simulink model "VM_22042020"  (R2019b)
settings: Solver=VariableStepAuto  StartTime=0.0  StopTime=120  RelTol=1e-3
libraries: aerolibconvert2 x3, simulink x2
settings Model: Creator=diego  LastModifiedBy=diego
settings DataIOCC: OutputOption=SpecifiedOutputTimes  OutputTimes=[0:0.0001:120]

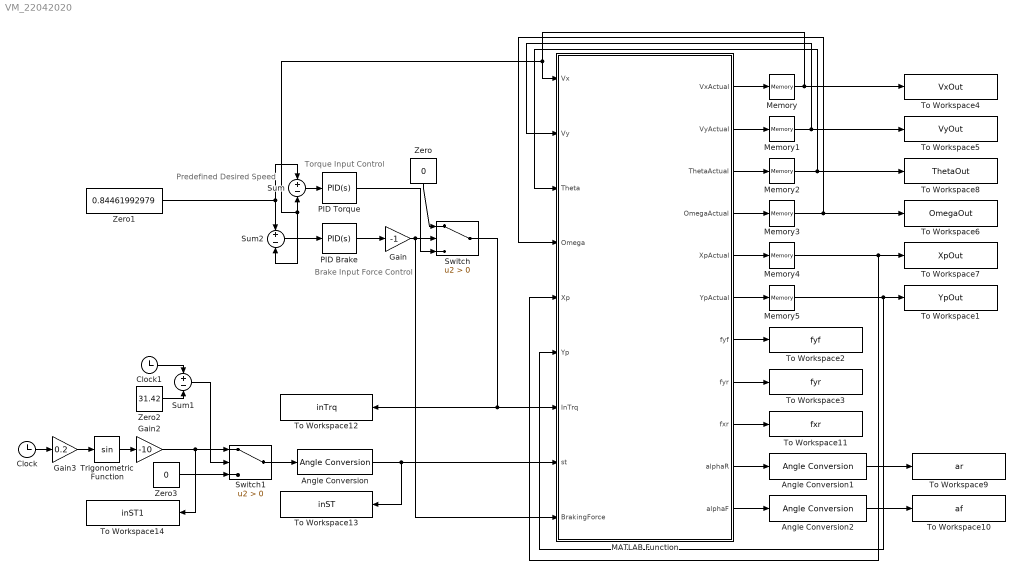
== system VM_22042020 ==
  note: Brake Input Force Control
  note: Torque Input Control
  note: Predefined Desired Speed
  Angle Conversion : aerolibconvert2/Angle Conversion  IU=deg  OU=rad
  Angle Conversion1 : aerolibconvert2/Angle Conversion  IU=rad  OU=deg
  Angle Conversion2 : aerolibconvert2/Angle Conversion  IU=rad  OU=deg
  Clock : Clock
  Clock1 : Clock
  Gain : Gain  Gain=-1
  Gain2 : Gain  Gain=-10
  Gain3 : Gain  Gain=0.2
  MATLAB Function : MATLAB Function  TreatAsAtomicUnit=on
  Memory{,1..5} (6 alike) : Memory
  PID Brake : simulink/Continuous/PID Controller  Controller=PID  Form=Parallel  TimeDomain=Continuous-time  SampleTime=-1  IntegratorMethod=Forward Euler  FilterMethod=Forward Euler  ControllerParametersSource=internal  P=7  I=0.28  D=0.5  UseFilter=on  N=100  TunerSelectOption=Transfer Function Based (PID Tuner App)  InitialConditionSource=internal  InitialConditionForIntegrator=0  InitialConditionForFilter=0  DifferentiatorICPrevScaledInput=0  ExternalReset=none  TrackingMode=off  Kt=1  LimitOutput=on  UpperSaturationLimit=0  LowerSaturationLimit=-10000  LinearizeAsGain=on  AntiWindupMode=none  Kb=1  POutMin=[]  POutMax=[]  IOutMin=[]  IOutMax=[]  DOutMin=[]  DOutMax=[]  NOutMin=[]  NOutMax=[]  SumOutMin=[]  SumOutMax=[]  SaturationOutMin=[]  SaturationOutMax=[]  PParamMin=[]  PParamMax=[]  IParamMin=[]  IParamMax=[]  DParamMin=[]  DParamMax=[]  NParamMin=[]  NParamMax=[]  KbParamMin=[]  KbParamMax=[]  KtParamMin=[]  KtParamMax=[]  KbOutMin=[]  KbOutMax=[]  KtOutMin=[]  KtOutMax=[]  IntegratorOutMin=[]  IntegratorOutMax=[]  FilterOutMin=[]  FilterOutMax=[]  SumI1OutMin=[]  SumI1OutMax=[]  SumI2OutMin=[]  SumI2OutMax=[]  SumI3OutMin=[]  SumI3OutMax=[]  SumI4OutMin=[]  SumI4OutMax=[]  SumDOutMin=[]  SumDOutMax=[]  DifferentiatorOutMin=[]  DifferentiatorOutMax=[]  FilterDiffOutCoefMin=[]  FilterDiffOutCoefMax=[]  ReciprocalOutMin=[]  ReciprocalOutMax=[]  SumDenOutMin=[]  SumDenOutMax=[]  SumNumOutMin=[]  SumNumOutMax=[]  DivideOutMin=[]  DivideOutMax=[]  IntegratorContinuousStateAttributes=''  IntegratorStateMustResolveToSignalObject=off  IntegratorRTWStateStorageClass=Auto  FilterContinuousStateAttributes=''  FilterStateMustResolveToSignalObject=off  FilterRTWStateStorageClass=Auto  ParallelPVariant=InternalParameters  IdealPVariant=Disabled  IVariant=InternalParameters  DVariant=InternalParameters  IntegratorVariant=Continuous  SatVariant=Enabled  AWVariant=Passthrough  PCopyVariant=Disabled  TRVariant=Disabled  FdbkBlocksVariant=Forward  IdealPFdbkVariant=Disabled  SatFdbkVariant=Disabled  DerivativeFilterVariant=ContFilter  NVariant=InternalParameters  NCopyVariant=Disabled  FilterICVariant=InternalICsFilter  IntegratorICVariant=InternalICs  ExternalResetVariant=Disabled  TRSumVariant=Passthrough  SumFdbkVariant=Disabled  SumVariant=Sum_PID
  PID Torque : simulink/Continuous/PID Controller  Controller=PID  Form=Parallel  TimeDomain=Continuous-time  SampleTime=-1  IntegratorMethod=Forward Euler  FilterMethod=Forward Euler  ControllerParametersSource=internal  P=12  I=0.5  D=0.5  UseFilter=on  N=100  TunerSelectOption=Transfer Function Based (PID Tuner App)  InitialConditionSource=internal  InitialConditionForIntegrator=0  InitialConditionForFilter=0  DifferentiatorICPrevScaledInput=0  ExternalReset=none  TrackingMode=off  Kt=1  LimitOutput=on  UpperSaturationLimit=120  LowerSaturationLimit=0  LinearizeAsGain=on  AntiWindupMode=none  Kb=1  POutMin=[]  POutMax=[]  IOutMin=[]  IOutMax=[]  DOutMin=[]  DOutMax=[]  NOutMin=[]  NOutMax=[]  SumOutMin=[]  SumOutMax=[]  SaturationOutMin=[]  SaturationOutMax=[]  PParamMin=[]  PParamMax=[]  IParamMin=[]  IParamMax=[]  DParamMin=[]  DParamMax=[]  NParamMin=[]  NParamMax=[]  KbParamMin=[]  KbParamMax=[]  KtParamMin=[]  KtParamMax=[]  KbOutMin=[]  KbOutMax=[]  KtOutMin=[]  KtOutMax=[]  IntegratorOutMin=[]  IntegratorOutMax=[]  FilterOutMin=[]  FilterOutMax=[]  SumI1OutMin=[]  SumI1OutMax=[]  SumI2OutMin=[]  SumI2OutMax=[]  SumI3OutMin=[]  SumI3OutMax=[]  SumI4OutMin=[]  SumI4OutMax=[]  SumDOutMin=[]  SumDOutMax=[]  DifferentiatorOutMin=[]  DifferentiatorOutMax=[]  FilterDiffOutCoefMin=[]  FilterDiffOutCoefMax=[]  ReciprocalOutMin=[]  ReciprocalOutMax=[]  SumDenOutMin=[]  SumDenOutMax=[]  SumNumOutMin=[]  SumNumOutMax=[]  DivideOutMin=[]  DivideOutMax=[]  IntegratorContinuousStateAttributes=''  IntegratorStateMustResolveToSignalObject=off  IntegratorRTWStateStorageClass=Auto  FilterContinuousStateAttributes=''  FilterStateMustResolveToSignalObject=off  FilterRTWStateStorageClass=Auto  ParallelPVariant=InternalParameters  IdealPVariant=Disabled  IVariant=InternalParameters  DVariant=InternalParameters  IntegratorVariant=Continuous  SatVariant=Enabled  AWVariant=Passthrough  PCopyVariant=Disabled  TRVariant=Disabled  FdbkBlocksVariant=Forward  IdealPFdbkVariant=Disabled  SatFdbkVariant=Disabled  DerivativeFilterVariant=ContFilter  NVariant=InternalParameters  NCopyVariant=Disabled  FilterICVariant=InternalICsFilter  IntegratorICVariant=InternalICs  ExternalResetVariant=Disabled  TRSumVariant=Passthrough  SumFdbkVariant=Disabled  SumVariant=Sum_PID
  Sum : Sum  Inputs=+-
  Sum1 : Sum  Inputs=+-
  Sum2 : Sum  Inputs=+-
  Switch : Switch  Criteria=u2 > Threshold
  Switch1 : Switch  Criteria=u2 > Threshold
  To Workspace1 : ToWorkspace  VariableName=YpOut  SaveFormat=Timeseries  SampleTime=-1
  To Workspace10 : ToWorkspace  VariableName=af  SaveFormat=Timeseries  SampleTime=-1
  To Workspace11 : ToWorkspace  VariableName=fxr  SaveFormat=Timeseries  SampleTime=-1
  To Workspace12 : ToWorkspace  VariableName=inTrq  SaveFormat=Timeseries  SampleTime=-1
  To Workspace13 : ToWorkspace  VariableName=inST  SaveFormat=Timeseries  SampleTime=-1
  To Workspace14 : ToWorkspace  VariableName=inST1  SaveFormat=Timeseries  SampleTime=-1
  To Workspace2 : ToWorkspace  VariableName=fyf  SaveFormat=Timeseries  SampleTime=-1
  To Workspace3 : ToWorkspace  VariableName=fyr  SaveFormat=Timeseries  SampleTime=-1
  To Workspace4 : ToWorkspace  VariableName=VxOut  SaveFormat=Timeseries  SampleTime=-1
  To Workspace5 : ToWorkspace  VariableName=VyOut  SaveFormat=Timeseries  SampleTime=-1
  To Workspace6 : ToWorkspace  VariableName=OmegaOut  SaveFormat=Timeseries  SampleTime=-1
  To Workspace7 : ToWorkspace  VariableName=XpOut  SaveFormat=Timeseries  SampleTime=-1
  To Workspace8 : ToWorkspace  VariableName=ThetaOut  SaveFormat=Timeseries  SampleTime=-1
  To Workspace9 : ToWorkspace  VariableName=ar  SaveFormat=Timeseries  SampleTime=-1
  Trigonometric Function : Trigonometry
  Zero : Constant  Value=0  OutDataTypeStr=Inherit: Inherit via back propagation
  Zero1 : Constant  Value=0.84461992979  OutDataTypeStr=Inherit: Inherit via back propagation
  Zero2 : Constant  Value=31.42  OutDataTypeStr=Inherit: Inherit via back propagation
  Zero3 : Constant  Value=0  OutDataTypeStr=Inherit: Inherit via back propagation
  wires:
  MATLAB Function/1(VxActual) -> Memory/1
  MATLAB Function/2(VyActual) -> Memory1/1
  MATLAB Function/3(ThetaActual) -> Memory2/1
  MATLAB Function/4(OmegaActual) -> Memory3/1
  MATLAB Function/5(XpActual) -> Memory4/1
  MATLAB Function/6(YpActual) -> Memory5/1
  Memory/1 -> To Workspace4/1, Sum2/2, Sum/2, MATLAB Function/1(Vx)
  Memory1/1 -> To Workspace5/1, MATLAB Function/2(Vy)
  Memory2/1 -> To Workspace8/1, MATLAB Function/3(Theta)
  Memory3/1 -> To Workspace6/1, MATLAB Function/4(Omega)
  Memory4/1 -> MATLAB Function/5(Xp), To Workspace7/1
  Memory5/1 -> MATLAB Function/6(Yp), To Workspace1/1
  Sum/1 -> PID Torque/1
  PID Brake/1 -> Gain/1
  Gain/1 -> MATLAB Function/9(BrakingForce), Switch/2
  Zero1/1 -> Sum/1, Sum2/1
  PID Torque/1 -> Switch/3
  Sum2/1 -> PID Brake/1
  Zero/1 -> Switch/1
  Switch/1 -> To Workspace12/1, MATLAB Function/7(InTrq)
  MATLAB Function/7(fyf) -> To Workspace2/1
  MATLAB Function/8(fyr) -> To Workspace3/1
  MATLAB Function/9(fxr) -> To Workspace11/1
  Angle Conversion/1 -> MATLAB Function/8(st), To Workspace13/1
  MATLAB Function/10(alphaR) -> Angle Conversion1/1
  Angle Conversion1/1 -> To Workspace9/1
  MATLAB Function/11(alphaF) -> Angle Conversion2/1
  Angle Conversion2/1 -> To Workspace10/1
  Switch1/1 -> Angle Conversion/1
  Trigonometric Function/1 -> Gain2/1
  Clock/1 -> Gain3/1
  Zero3/1 -> Switch1/3
  Gain2/1 -> To Workspace14/1, Switch1/1
  Clock1/1 -> Sum1/1
  Zero2/1 -> Sum1/2
  Sum1/1 -> Switch1/2
  Gain3/1 -> Trigonometric Function/1

== matlab function VM_22042020/MATLAB Function ==
  data: Vx input; VxActual output; Vy input; Theta input; Omega input; Xp input; Yp input; InTrq input; st input; BrakingForce input; VyActual output; ThetaActual output; OmegaActual output; XpActual output; YpActual output; fyf output; fyr output; fxr output; alphaR output; alphaF output
function [VxActual,VyActual,ThetaActual,OmegaActual,XpActual,YpActual,fyf,fyr,fxr,alphaR,alphaF] = VehicleModel(Vx,Vy,Theta,Omega,Xp,Yp,InTrq,st,BrakingForce)
%Center of gravity location from vehicle rear axle
Lf =0.669670;
%Rear axle to center of gravity distance
Lr = 0.669670;
%Total lenght
L =Lf + Lr;
%Vehicle mas 
m = 400;
%Gravity
g = 9.81;
%weight
W = g*m;
%Friction Coef.
miu = 0.9;
%height of the center of gravity
hgc = 0.38;
%Wheel r
rad = 0.2876;
%height
height = 0.4052;
%width 
w = 1.1600;
%Vehicle yaw inertia
I = 1/12 *m*(w^2+height^2);


%Force values
fxr = InTrq/rad + BrakingForce;
fxf = 0;

%The vertical force acting on a tire
fzr = (m*g*Lf)/L + (fxr*hgc)/(L);
fzf = (m*g*Lr)/L - (fxr*hgc)/(L);

%Validating initial conditions
if(Vx ==0)
    alphaR = 0;
    alphaF = 0;
else
    alphaR = (Lr*Omega-Vy)/Vx;
    alphaF = st-(Lf*Omega+Vy)/Vx;
end

if(isnan(alphaR))
    alphaR = 0;
end

if(isnan(alphaF))
    alphaF = 0;
end

C = 1.49;
B = 0.244;
E = 0;

sh =0;
sv =0;
xf = alphaF + sh;
xr = alphaR + sh;

fyf = fzf*sin( C*atan(B*xf - E*(B*xf - atan(B*xf))) ) + sv;
fyr = fzr*sin( C*atan(B*xr - E*(B*xr - atan(B*xr))) ) + sv;

%VehicleModel
VxActual = (fxf * cos(st) + fxr - fyf*sin(st))/m + Vy*Omega;
VyActual = (fyr + fyf*cos(st)+fxf*sin(st))/m - Vx*Omega;
OmegaActual = (Lf*fyf*cos(st)-Lr*fyr+Lf*fxf*sin(st))/I;
ThetaActual = Omega;
XpActual = Vx*cos(2*pi-Theta)+Vy*cos(3/4*pi-Theta);
YpActual = Vx*sin(2*pi-Theta)+Vy*sin(3/4*pi-Theta);

%Runge Kutta Fourth Order
%x0 - Theta (Yaw Angle)
%x1 - Omega (Yaw Rate)
%x2 - Lateral Velocity Vy
%x3 - Longitudinal Velocity Vx
%x4 - Global X position
%x5 - Global Y position

%Time Step
h = 0.0001;

x0 = Theta;
x1 = Omega;
x2 = Vy;
x3 = Vx;
x4 = Xp;
x5 = Yp;

k00 = h*x0dot(x1);
k10 = h*x1dot(Lf,fxf,st,Lr,fyf,fyr,I);
k20 = h*x2dot(fxf,st,fyf,fyr,x3,x1,m);
k30 = h*x3dot(fxf,fxr,fyf,st,x2,x1,m);
k40 = h*x4dot(x2,x0,x3);
k50 = h*x5dot(x2,x0,x3);

k01 = h*x0dot(x1+0.5*k10);
k11 = h*x1dot(Lf,fxf,st,Lr,fyf,fyr,I);
k21 = h*x2dot(fxf,st,fyf,fyr,x3+0.5*k30, x1+0.5*k10,m);
k31 = h*x3dot(fxf,fxr,fyf,st,x2+0.5*k20, x1+0.5*k10,m);
k41 = h*x4dot(x2+0.5*k20,x0+0.5*k00,x3+0.5*k30);
k51 = h*x5dot(x2+0.5*k20,x0+0.5*k00,x3+0.5*k30);

k02 = h*x0dot(x1+0.5*k11);
k12 = h*x1dot(Lf,fxf,st,Lr,fyf,fyr,I);
k22 = h*x2dot(fxf,st,fyf,fyr,x3+0.5*k31, x1+0.5*k11,m);
k32 = h*x3dot(fxf,fxr,fyf,st,x2+0.5*k21, x1+0.5*k11,m);
k42 = h*x4dot(x2+0.5*k21,x0+0.5*k01,x3+0.5*k31);
k52 = h*x5dot(x2+0.5*k21,x0+0.5*k01,x3+0.5*k31);

k03 = h*x0dot(x1+k12);
k13 = h*x1dot(Lf,fxf,st,Lr,fyf,fyr,I);
k23 = h*x2dot(fxf,st,fyf,fyr,x3+k32, x1+k12,m);
k33 = h*x3dot(fxf,fxr,fyf,st,x2+k22, x1+k12,m);
k43 = h*x4dot(x2+k22,x0+k02,x3+k32);
k53 = h*x5dot(x2+k22,x0+k02,x3+k32);

ThetaActual = x0+1/6*(k00+2*k01+2*k02+k03);
OmegaActual = x1+1/6*(k10+2*k11+2*k12+k13);
VyActual = x2+1/6*(k20+2*k21+2*k22+k23);
VxActual = x3+1/6*(k30+2*k31+2*k32+k33);
XpActual = x4+1/6*(k40+2*k41+2*k42+k43);
YpActual = x5+1/6*(k50+2*k51+2*k52+k53);
